simulink model "TD1_Ex2_model"  (R2022a)
settings: Solver=VariableStepAuto  StartTime=0.0  StopTime=10  MaxStep=0.1  RelTol=1e-3
undefined symbols (not defined in the file): A, B, u0, x0, x0_lin, x_eq
settings Model: Creator=aranovskiy_sta  LastModifiedBy=CS

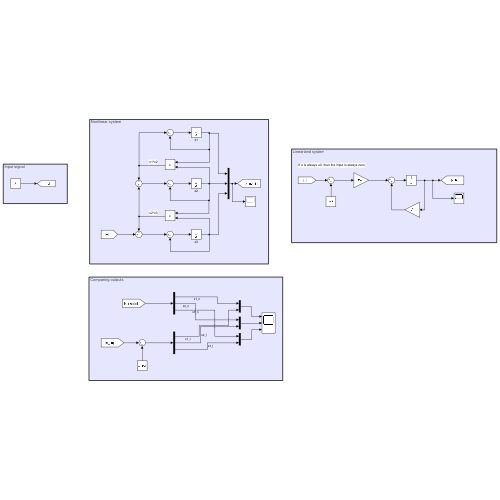
[thumbnail: Simulink's stored preview of the top-level diagram]
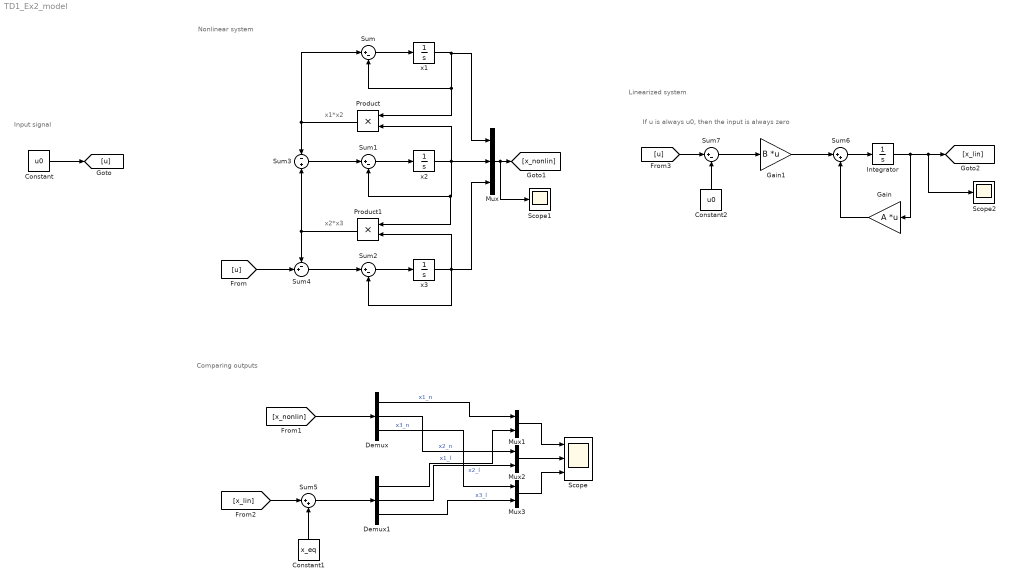
== system TD1_Ex2_model ==
  note: If u is always u0, then the input is always zero
  note: Comparing outputs
  note: Linearized system
  note: Nonlinear system
  note: Input signal
  note: x2*x3
  note: x1*x2
  Constant : Constant  Value=u0
  Constant1 : Constant  Value=x_eq
  Constant2 : Constant  Value=u0
  Demux : Demux  Outputs=3
  Demux1 : Demux  Outputs=3
  Gain : Gain  Gain=A  Multiplication=Matrix(K*u)
  Gain1 : Gain  Gain=B  Multiplication=Matrix(K*u)
  Integrator : Integrator  InitialCondition=x0_lin
  Mux : Mux  Inputs=3
  Mux1 : Mux  Inputs=2
  Mux2 : Mux  Inputs=2
  Mux3 : Mux  Inputs=2
  Product : Product
  Product1 : Product
  Scope : Scope  NumInputPorts=3
  Scope1 : Scope
  Scope2 : Scope
  Sum{,1..2,7} (4 alike) : Sum  Inputs=|+-
  Sum3 : Sum  Inputs=-+
  Sum4 : Sum  Inputs=-+|
  Sum5 : Sum  Inputs=|++
  Sum6 : Sum  Inputs=|++
  x1 : Integrator  InitialCondition=x0(1)
  x2 : Integrator  InitialCondition=x0(2)
  x3 : Integrator  InitialCondition=x0(3)
  wires:
  x1/1 -> Product/1, Sum/2, Mux/1
  Sum/1 -> x1/1
  Sum1/1 -> x2/1
  x2/1 -> Mux/2, Product/2, Product1/1, Sum1/2
  x3/1 -> Mux/3, Sum2/2, Product1/2
  Sum2/1 -> x3/1
  Product/1 -> Sum3/1, Sum/1
  Product1/1 -> Sum4/1, Sum3/2
  Sum3/1 -> Sum1/1
  Sum4/1 -> Sum2/1
  [u] -> Sum4/2
  Constant/1 -> [u]
  Integrator/1 -> Scope2/1, [x_lin], Gain/1
  Mux/1 -> Scope1/1, [x_nonlin]
  [x_lin] -> Sum5/1
  Constant1/1 -> Sum5/2
  [x_nonlin] -> Demux/1
  Sum5/1 -> Demux1/1
  Demux/1 -> Mux1/1  "x1_n"
  Demux1/1 -> Mux1/2  "x1_l"
  Demux/2 -> Mux2/1  "x2_n"
  Demux1/2 -> Mux2/2  "x2_l"
  Demux/3 -> Mux3/1  "x3_n"
  Demux1/3 -> Mux3/2  "x3_l"
  Mux2/1 -> Scope/2
  Mux1/1 -> Scope/1
  Mux3/1 -> Scope/3
  Sum6/1 -> Integrator/1
  Gain/1 -> Sum6/2
  Gain1/1 -> Sum6/1
  [u] -> Sum7/1
  Constant2/1 -> Sum7/2
  Sum7/1 -> Gain1/1
